simulink model "Simulink_Monomotor"  (R2023b)
settings: Solver=ode45  StartTime=0.0  StopTime=120  RelTol=1e-3  EnableMultiTasking=on
values from neighbouring files (symbols this model uses):
  g = 9.8    [Code_Monomotor.m]
  Jb = 7.5e-3    (= 0.0075)    [Code_Monomotor.m]
  JM = 4.987e-6    (= 4.987e-06)    [Code_Monomotor.m]
  Ke = 5.372e-3    (= 0.005372)    [Code_Monomotor.m]
  Kf = Kt*Ke/R    (= 0.000456023111111)    [Code_Monomotor.m]
  Kq = Cd*rho*(D^5)/(4*pi^2)    (= 3.00837911482e-07)    [Code_Monomotor.m]
  Ks = Ct*rho*(D^4)/(4*pi^2)    (= 1.24114706163e-05)    [Code_Monomotor.m]
  Kt = 7.64e-3    (= 0.00764)    [Code_Monomotor.m]
  l = 0.3    [Code_Monomotor.m]
  L = 0.1e-3    (= 0.0001)    [Code_Monomotor.m]
  M = 0.052    [Code_Monomotor.m]
  R = 0.09    [Code_Monomotor.m]
libraries: fuzblock x1, slpidlib x1
settings Model: Creator=User  LastModifiedBy=vscon
settings SolverCC: AlgebraicLoopSolver=TrustRegion
settings DataIOCC: LimitDataPoints=on  SaveFormat=Array  ReturnWorkspaceOutputs=off
settings OptimizationCC: LifeSpan=inf
settings DebuggingCC: SolverPrmCheckMsg=warning  UnconnectedInputMsg=warning  UnconnectedOutputMsg=warning  UnconnectedLineMsg=warning  SFUnexpectedBacktrackingDiag=warning  SFNoUnconditionalDefaultTransitionDiag=warning  SFExecutionAtInitializationDiag=none  ArithmeticOperatorsInVariantConditions=warning
settings HardwareCC: ProdBitPerPointer=32  ProdBitPerSizeT=32  ProdBitPerPtrDiffT=32  ProdLargestAtomicFloat=None  ProdIntDivRoundTo=Undefined  ProdEndianess=Unspecified  ProdWordSize=32  ProdHWDeviceType=32-bit Generic
settings ModelReferenceCC: PropagateSignalLabelsOutOfModel=off
settings SFSimCC: SimUseLocalCustomCode=off  CustomCodeUndefinedFunction=UseInterfaceOnly
settings RTWCC: RTWUseLocalCustomCode=off
settings CodeAppCC: StateflowObjectComments=on
settings GRTTargetCC: TargetLangStandard=C89/C90 (ANSI)
settings ConfigComp: CovMetricSettings=dw  CovSaveCumulativeToWorkspaceVar=on  CovSaveSingleToWorkspaceVar=on  CovExternalEMLEnable=off  CovSFcnEnable=off

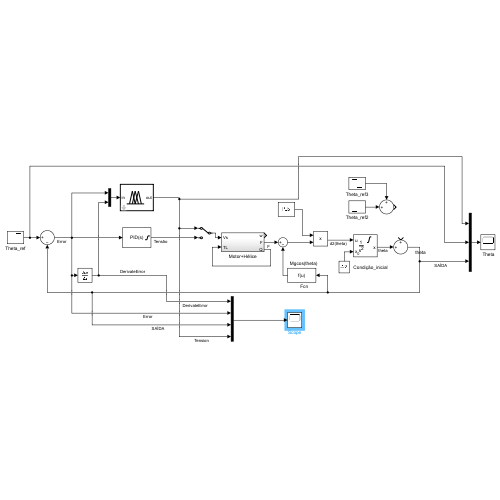
[thumbnail: Simulink's stored preview of the top-level diagram]
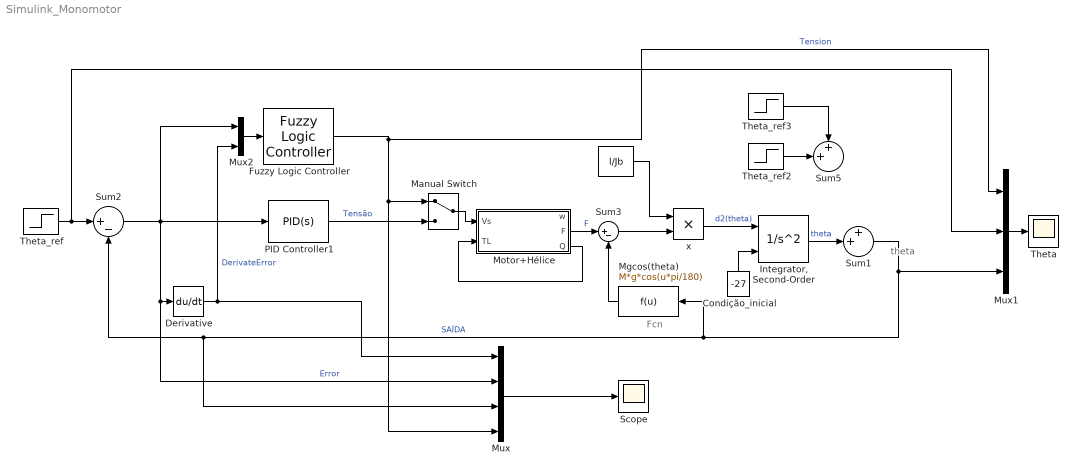
== system Simulink_Monomotor ==
  note: theta
  note: Fcn
  "  " : Constant  Value=l/Jb
  "   Mgcos(theta)" : Fcn  Expr=M*g*cos(u*pi/180)
  " Condição_inicial" : Constant  Value=-27  VectorParams1D=off
  " Theta" : Scope
  Derivative : Derivative
  Fuzzy Logic Controller : fuzblock/Fuzzy Logic  Controller  FIS=fuzzyFIS  OutputSampleNumber=101  DataType=double  FuzzifiedInputs=off  RuleFiringStrengths=off  RuleOutputs=off  AggregatedOutputs=off  SimulateUsing=Interpreted execution  OutOfRangeInputValueMessage=warning  NoRuleFiredMessage=warning  EmptyOutputFuzzySetMessage=warning
  "Integrator, Second-Order" : SecondOrderIntegrator  ICSourceX=external  LimitX=on  UpperLimitX=27  LowerLimitX=-27  ShowOutput=x
  Manual Switch : ManualSwitch
  Motor+Hélice : Subsystem
  Mux : Mux
  Mux1 : Mux  Inputs=3
  Mux2 : Mux  Inputs=2
  PID Controller1 : slpidlib/PID Controller  Controller=PID  Form=Parallel  TimeDomain=Continuous-time  UseExternalTs=off  SampleTime=1  IntegratorMethod=Forward Euler  FilterMethod=Forward Euler  ControllerParametersSource=internal  P=0.1  I=0.03  UseKiTs=off  D=0.1  N=100  UseFilter=on  TunerSelectOption=Transfer Function Based (PID Tuner App)  InitialConditionSource=internal  InitialConditionForIntegrator=0  InitialConditionForFilter=0  DifferentiatorICPrevScaledInput=0  ExternalReset=none  TrackingMode=off  Kt=1  LimitOutput=on  SatLimitsSource=internal  UpperSaturationLimit=10  LowerSaturationLimit=0  LinearizeAsGain=off  AntiWindupMode=back-calculation  Kb=1  LimitIntegrator=off  UpperIntegratorSaturationLimit=inf  LowerIntegratorSaturationLimit=-inf  POutMin=[]  POutMax=[]  IOutMin=[]  IOutMax=[]  DOutMin=[]  DOutMax=[]  NOutMin=[]  NOutMax=[]  SumOutMin=[]  SumOutMax=[]  SaturationOutMin=[]  SaturationOutMax=[]  PParamMin=[]  PParamMax=[]  IParamMin=[]  IParamMax=[]  DParamMin=[]  DParamMax=[]  NParamMin=[]  NParamMax=[]  KbParamMin=[]  KbParamMax=[]  KtParamMin=[]  KtParamMax=[]  KbOutMin=[]  KbOutMax=[]  KtOutMin=[]  KtOutMax=[]  IntegratorOutMin=[]  IntegratorOutMax=[]  FilterOutMin=[]  FilterOutMax=[]  SumI1OutMin=[]  SumI1OutMax=[]  SumI2OutMin=[]  SumI2OutMax=[]  SumI3OutMin=[]  SumI3OutMax=[]  SumI4OutMin=[]  SumI4OutMax=[]  SumDOutMin=[]  SumDOutMax=[]  DifferentiatorOutMin=[]  DifferentiatorOutMax=[]  FilterDiffOutCoefMin=[]  FilterDiffOutCoefMax=[]  ReciprocalOutMin=[]  ReciprocalOutMax=[]  SumDenOutMin=[]  SumDenOutMax=[]  SumNumOutMin=[]  SumNumOutMax=[]  DivideOutMin=[]  DivideOutMax=[]  UdiffTsProdOutMin=[]  UdiffTsProdOutMax=[]  NTsProdOutMin=[]  NTsProdOutMax=[]  UintegralTsProdOutMin=[]  UintegralTsProdOutMax=[]  UngainTsProdOutMin=[]  UngainTsProdOutMax=[]  ClampingZeroOutDataTypeStr=Inherit: Inherit via back propagation  ClampingZeroOutMin=[]  ClampingZeroOutMax=[]  FilterDenConstantOutDataTypeStr=Inherit: Inherit via back propagation  FilterDenConstantOutMin=[]  FilterDenConstantOutMax=[]  PCopyOutDataTypeStr=Inherit: Inherit via back propagation  PCopyOutMin=[]  PCopyOutMax=[]  NCopyOutDataTypeStr=Inherit: Inherit via back propagation  NCopyOutMin=[]  NCopyOutMax=[]  IntegratorContinuousStateAttributes=''  IntegratorStateMustResolveToSignalObject=off  IntegratorRTWStateStorageClass=Auto  FilterContinuousStateAttributes=''  FilterStateMustResolveToSignalObject=off  FilterRTWStateStorageClass=Auto  ParallelPVariant=InternalParameters  IdealPVariant=Disabled  IVariant=InternalParameters  DVariant=InternalParameters  IntegratorVariant=Continuous  SatVariant=Enabled  AWVariant=BackCalculation  PCopyVariant=Disabled  TRVariant=Disabled  FdbkBlocksVariant=Forward  IdealPFdbkVariant=Disabled  SatFdbkVariant=Disabled  DerivativeFilterVariant=ContFilter  NVariant=InternalParameters  NCopyVariant=Disabled  FilterICVariant=InternalICsFilter  IntegratorICVariant=InternalICs  ExternalResetVariant=Disabled  TRSumVariant=Passthrough  SumFdbkVariant=Disabled  SumVariant=Sum_PID  TsampFilterVariant=InternalTs  TsampNgainVariant=Passthrough  TsampIntegralVariant=Disabled_SignalSpec  ExternalSaturationOutDataTypeStr=Inherit: Same as second input
  Scope : Scope
  Sum1 : Sum  Inputs=++|
  Sum2 : Sum  Inputs=|+-
  Sum3 : Sum  Inputs=|+-
  Sum5 : Sum  Inputs=++|
  Theta_ref : Step  Time=0  After=0  SampleTime=0  ZeroCross=off
  Theta_ref2 : Step  Time=43  After=15  SampleTime=0  ZeroCross=off
  Theta_ref3 : Step  Time=40  After=-15  SampleTime=0  ZeroCross=off
  x : Product
  wires:
  "  "/1 -> x/1
  Sum3/1 -> x/2
  x/1 -> "Integrator, Second-Order"/1  "d2(theta)"
  Mux1/1 -> " Theta"/1
  Theta_ref/1 -> Mux1/2, Sum2/1
  " Condição_inicial"/1 -> "Integrator, Second-Order"/2
  Motor+Hélice/2(F) -> Sum3/1  "F"
  Motor+Hélice/3(Q) -> Motor+Hélice/2(TL)
  "   Mgcos(theta)"/1 -> Sum3/2
  Sum1/1 -> "   Mgcos(theta)"/1, Mux/3, Sum2/2, Mux1/3  "SAÍDA"
  "Integrator, Second-Order"/1 -> Sum1/2  "theta"
  Theta_ref3/1 -> Sum5/1
  Theta_ref2/1 -> Sum5/2
  Sum2/1 -> Mux2/1, Mux/2, Derivative/1, PID Controller1/1  "Error"
  Derivative/1 -> Mux/1, Mux2/2  "DerivateError"
  Mux/1 -> Scope/1
  Fuzzy Logic Controller/1 -> Mux1/1, Mux/4, Manual Switch/1  "Tension"
  Mux2/1 -> Fuzzy Logic Controller/1
  Manual Switch/1 -> Motor+Hélice/1(Vs)
  PID Controller1/1 -> Manual Switch/2  "Tensão"

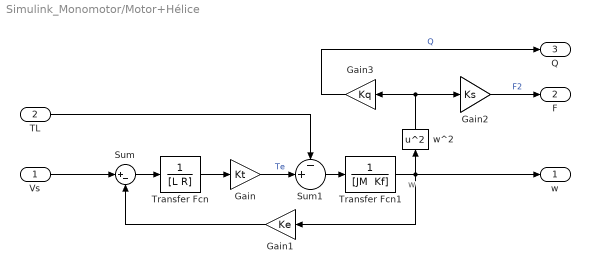
== system Simulink_Monomotor/Motor+Hélice ==
  note: w
  Vs : Inport
  TL : Inport  Port=2
  Gain : Gain  Gain=Kt
  Gain1 : Gain  Gain=Ke
  Gain2 : Gain  Gain=Ks
  Gain3 : Gain  Gain=Kq
  Sum : Sum  Inputs=|+-
  Sum1 : Sum  Inputs=-+|
  Transfer Fcn : TransferFcn  Denominator=[L R]
  Transfer Fcn1 : TransferFcn  Denominator="[JM  Kf]"
  w^2 : Fcn  Expr=u^2
  w : Outport
  F : Outport  Port=2
  Q : Outport  Port=3
  wires:
  TL/1 -> Sum1/1
  Gain3/1 -> Q/1  "Q"
  Vs/1 -> Sum/1
  Transfer Fcn1/1 -> w/1, w^2/1, Gain1/1
  Gain1/1 -> Sum/2
  Sum1/1 -> Transfer Fcn1/1
  Gain/1 -> Sum1/2  "Te"
  Transfer Fcn/1 -> Gain/1
  Sum/1 -> Transfer Fcn/1
  Gain2/1 -> F/1  "F2"
  w^2/1 -> Gain2/1, Gain3/1
